simulink model "pruba_mex_s_funkcij"  (R2017a)
settings: Solver=VariableStepAuto  StartTime=0.0  StopTime=10  RelTol=1e-3
settings Model: Creator=Szwank  LastModifiedBy=Szwank

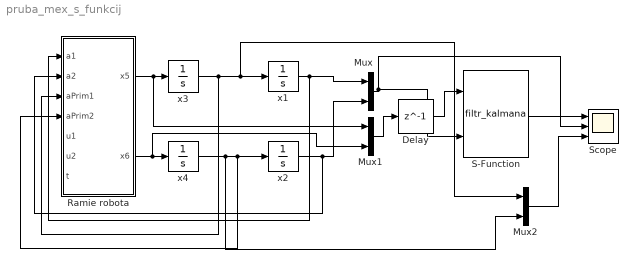
== system pruba_mex_s_funkcij ==
  Delay : Delay  DelayLength=1  InitialCondition=0
  Mux : Mux  Inputs=2
  Mux1 : Mux  Inputs=2
  Mux2 : Mux  Inputs=2
  Ramie robota : MATLAB Function  TreatAsAtomicUnit=on
  S-Function : S-Function  FunctionName=filtr_kalmana  Parameters=[-(pi/2)-0.3; 0.3; 0; 0]  SFunctionDeploymentMode=off  EnableBusSupport=off
  Scope : Scope  NumInputPorts=3
  x1 : Integrator  InitialCondition=-(pi/2)-0.3  AbsoluteTolerance=1e-5
  x2 : Integrator  InitialCondition=0.3  AbsoluteTolerance=1e-5
  x3 : Integrator  AbsoluteTolerance=1e-5
  x4 : Integrator  AbsoluteTolerance=1e-5
  wires:
  S-Function/1 -> Scope/1
  x3/1 -> Ramie robota/3(aPrim1), Mux2/1, x1/1
  Ramie robota/1(x5) -> Mux1/1, x3/1
  x4/1 -> Mux2/2, Ramie robota/4(aPrim2), x2/1
  Ramie robota/2(x6) -> Mux1/2, x4/1
  x1/1 -> Ramie robota/1(a1), Mux/1
  x2/1 -> Ramie robota/2(a2), Mux/2
  Mux/1 -> S-Function/2, Scope/2
  Mux2/1 -> Scope/3
  Delay/1 -> S-Function/1
  Mux1/1 -> Delay/1

== matlab function pruba_mex_s_funkcij/Ramie robota ==
  data: a1 input; a2 input; aPrim1 input; aPrim2 input; u1 input; u2 input; x5 output; x6 output; t input
function [x5,x6] = fcn(a1,a2,aPrim1,aPrim2,u1,u2,t)
m1 = 2; m2 = 1 * 1.15; l1 = 1.5; l2 = 1; lc1 = l1/2; lc2 = l2/2; J1 = (m1*l1^2)/3; J2 = (m2*l2^2)/3; g = 9.81;
H11 = m1*lc1^2 + J1 + m2*(l1^2 + lc2^2 + 2*l1*l2*cos(a2)) + J2;
H12  = m2*l1*lc2*cos(a2) + m2*lc2^2 + J2;
H21 = H12;
H22 = m2*lc2^2 + J2;
h = m2*l1*lc2*sin(a2);
g1 = m1*lc1*g*cos(a1) + m2*g*(lc2*cos(a1+a2)+l1*cos(a1));
g2 = m2*lc2*g*cos(a1+a2);
H = [H11 H12; H21 H22];
H2 = inv(H);
Z = [0;0];

J = [-h*aPrim2, -h*aPrim1-h*aPrim2; h*aPrim1,0];
M = [g1;g2];
U = [u1;u2];
%rozwikłanie 
Roz = -1*H2*J*[aPrim1; aPrim2] -1*H2*M + H2*U + H2 * Z; 
x5 = Roz(1);
x6 = Roz(2);
% x5 = (200*T1 - 200*T2 + (2943*cos(x1 + 2*x2))/2 - (8829*cos(x1))/2 + 150*x3^2*sin(x2) + 150*x4^2*sin(x2) + 225*x3^2*sin(2*x2) - 23544*J2*cos(x1) - 600*T2*cos(x2) + 800*J2*T1 - 800*J2*T2 + 300*x3*x4*sin(x2) + 600*J2*x3^2*sin(x2) + 600*J2*x4^2*sin(x2) + 1200*J2*x3*x4*sin(x2))/(25*(8*J1 + 108*J2 - 9*cos(2*x2) + 32*J1*J2 + 18));
% x6 = -(400*T1 - 5800*T2 - 17658*cos(x1 - x2) + 2943*cos(x1 + 2*x2) + 8829*cos(x1 + x2) - 8829*cos(x1) + 4350*x3^2*sin(x2) + 300*x4^2*sin(x2) + 7848*J1*cos(x1 + x2) + 900*x3^2*sin(2*x2) + 450*x4^2*sin(2*x2) - 47088*J2*cos(x1) + 1200*T1*cos(x2) - 2400*T2*cos(x2) - 1600*J1*T2 + 1600*J2*T1 - 1600*J2*T2 + 600*x3*x4*sin(x2) + 1200*J1*x3^2*sin(x2) + 1200*J2*x3^2*sin(x2) + 1200*J2*x4^2*sin(x2) + 900*x3*x4*sin(2*x2) + 2400*J2*x3*x4*sin(x2))/(50*(8*J1 + 108*J2 - 9*cos(2*x2) + 32*J1*J2 + 18));

%y = u;
